simulink model "sf_abs"  (R2017b)
settings: Solver=VariableStepDiscrete  StartTime=0.0  StopTime=20  MaxStep=.2  RelTol=1e-3  EnableMultiTasking=on
settings Model: ExtModeAutoUpdateStatusClock=off  Creator=The MathWorks, Inc.  LastModifiedBy=The MathWorks, Inc.
settings SolverCC: ZeroCrossControl=EnableAll  InsertRTBMode=Auto
settings DataIOCC: LimitDataPoints=on  SaveFormat=Array
settings OptimizationCC: ExpressionDepthLimit=2147483647  InitFltsAndDblsToZero=on  LifeSpan=inf
settings DebuggingCC: UnderspecifiedInitializationDetection=Classic  MergeDetectMultiDrivingBlocksExec=none  SignalResolutionControl=TryResolveAllWithWarning  SolverPrmCheckMsg=warning  FcnCallInpInsideContextMsg=warning  StateNameClashWarn=warning  StrictBusMsg=Warning  SFUnexpectedBacktrackingDiag=warning  SFNoUnconditionalDefaultTransitionDiag=warning  SFExecutionAtInitializationDiag=none
settings HardwareCC: ProdBitPerPointer=32  ProdBitPerSizeT=32  ProdBitPerPtrDiffT=32  ProdLargestAtomicFloat=None  ProdIntDivRoundTo=Undefined  ProdEndianess=Unspecified  ProdWordSize=32  ProdHWDeviceType=32-bit Generic
settings ModelReferenceCC: PropagateSignalLabelsOutOfModel=off
settings SFSimCC: SFSimEcho=off  SimParseCustomCode=off
settings CodeAppCC: StateflowObjectComments=on
settings GRTTargetCC: TargetFcnLib=ansi_tfl_tmw_new.mat  TargetLangStandard=C89/C90 (ANSI)  GeneratePreprocessorConditionals=Disable all  CombineOutputUpdateFcns=off  GRTInterface=on
settings ConfigComp: CovMetricSettings=dw  CovHtmlReporting=on  CovSaveCumulativeToWorkspaceVar=on  CovSaveSingleToWorkspaceVar=on  CovExternalEMLEnable=off  CovSFcnEnable=off

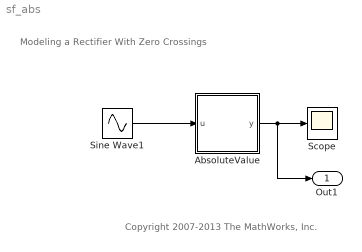
== system sf_abs ==
  note: Modeling a Rectifier With Zero Crossings
  note: Copyright 2007-2013 The MathWorks, Inc.
  AbsoluteValue : Stateflow chart  TreatAsAtomicUnit=on
  Scope : Scope
  Sine Wave1 : Sin  SampleTime=0
  Out1 : Outport
  wires:
  AbsoluteValue/1(y) -> Scope/1, Out1/1
  Sine Wave1/1 -> AbsoluteValue/1(u)

== stateflow chart sf_abs/AbsoluteValue ==
  settings: updateMethod=CONTINUOUS
  state N
    du: y = -u;
  state P
    du: y = u;
  (default) -> (junction 9)
  (junction 9) -> (junction 10) [order 2]
  (junction 10) -> N
  (junction 9) -> P [order 1] : [u >= 0]
  P -> N : [u < 0]
  N -> P : [u >= 0]
  data: u input; y output double
